simulink model "Driveline"  (R2020a)
settings: Solver=ode23tb  StartTime=0.0  StopTime=inf  FixedStep=.001  RelTol=1e-3
model workspace (MAT data in the model file):
  Trans.InputShaftInertia = 0.01
  Trans.InputShaftDamping = 0.001
  Trans.FinalDrive = 2.77
  Trans.GearRatios = [-3.82 4.56 4.56 2.97 2.08 1.69 1.27 1 0.85 0.65]
  Trans.GearNums = [-1 0 1 2 3 4 5 6 7 8]
  Trans.Inertias = [0.128 0.128 0.128 0.1 0.062 0.028 0.01 0.01 0.01 0.01]
  Trans.DampingCoeffs = [0.003 0.001 0.003 0.0025 0.002 0.001 0.001 0.001 0.001 0.001]
  Trans.Efficiencies = [0.9 0.9 0.9 0.9 0.9 0.95 0.95 0.95 0.95 0.95]
  Trans.ShiftTau = 0.02
  VEH.Mass = 330
  VEH.StaticNormalFrontLoad.FR = 74.25
  VEH.StaticNormalFrontLoad.FL = 74.25
  VEH.StaticNormalRearLoad.RR = 90.75
  VEH.StaticNormalRearLoad.RL = 90.75
  VEH.WheelBase = 1.575
  VEH.FrontAxlePositionfromCG = 0.847
  VEH.RearAxlePositionfromCG = 0.693
  VEH.HeightCG = 0.277
  VEH.FrontalArea = 1.435
  VEH.DragCoefficient = 0.33
  VEH.NumberOfWheelsPerAxle = 2
  VEH.Thread.FR = 1.705
  VEH.Thread.RR = 1.705
  VEH.PitchMomentInertia = 206
  VEH.RollMomentInertia = 206.613792
  VEH.YawMomentInertia = 206.613792
  VEH.SteeringRatio = 5.2
  VEH.TrackWidth = 1.2
  VEH.SprungMass = 290
  VEH.InitialLongPosition = 0
  VEH.InitialLatPosition = 0
  VEH.InitialVertPosition = 0
  VEH.InitialRollAngle = 0
  VEH.InitialPitchAngle = 0
  VEH.InitialYawAngle = 0
  VEH.InitialLongVel = 0
  VEH.InitialLatVel = 0
  VEH.InitialVertVel = 0
  VEH.InitialRollRate = 0
  VEH.InitialPitchRate = 0
  VEH.InitialYawRate = 0
  VEH.LongitudinalDragCoefficient = 1.06
  VEH.LongitudinalLCoefficient = -2.05
libraries: autolibsharedcoupling x4, vehdynlibsteering x1
settings Model: ModifiedByFormat=The MathWorks, Inc.  OrderedModelArguments=off  Creator=The MathWorks, Inc.  LastModifiedBy=The MathWorks, Inc.
settings SolverCC: ZeroCrossControl=DisableAll  DecoupledContinuousIntegration=on
settings DataIOCC: ReturnWorkspaceOutputs=off
settings DebuggingCC: ArtificialAlgebraicLoopMsg=none  IgnoredZcDiagnostic=none  PregeneratedLibrarySubsystemCodeDiagnostic=none  ArithmeticOperatorsInVariantConditions=warning
settings ModelReferenceCC: ModelReferenceMinAlgLoopOccurrences=on
settings SFSimCC: SimUseLocalCustomCode=off  CustomCodeUndefinedFunction=UseInterfaceOnly
settings RTWCC: RTWUseLocalCustomCode=off

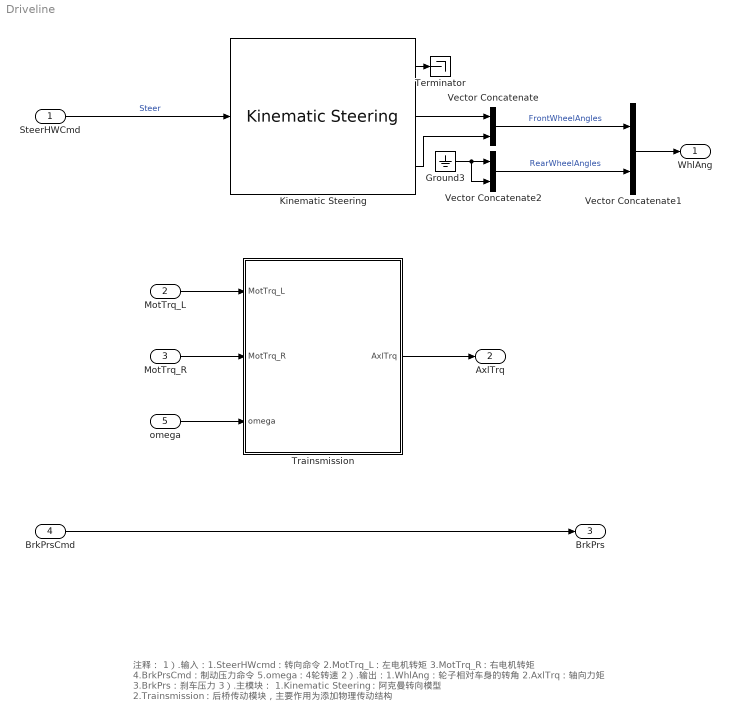
== system Driveline ==
  note: 注释：
      | 1）.输入：1.SteerHWcmd：转向命令
      | 2.MotTrq_L：左电机转矩
      | 3.MotTrq_R：右电机转矩
      | 4.BrkPrsCmd：制动压力命令
      | 5.omega：4轮转速
      | 2）.输出：1.WhlAng：轮子相对车身的转角
      | 2.AxlTrq：轴向力矩
      | 3.BrkPrs：刹车压力
      | 3）.主模块：
      | 1.Kinematic Steering：阿克曼转向模型
      | 2.Trainsmission：后桥传动模块，主要作用为添加物理传动结构
  SteerHWCmd : Inport
  MotTrq_L : Inport  Port=2
  MotTrq_R : Inport  Port=3
  BrkPrsCmd : Inport  Port=4  PortDimensions=4
  omega : Inport  Port=5
  Ground3 : Ground
  Kinematic Steering : vehdynlibsteering/Kinematic Steering  StrgType=Ackerman  StrgRatioType=Constant  Loc=Front  NrmlFctr=1  TrckWdth=VEH.WheelBase  WhlBase=(1.515+1.504)  Db=0  StrgRng=3*pi  StrgAngBpts="[-6.2832   -5.0265   -3.7699   -2.5133   -1.2566         0    1.2566    2.5133    3.7699    5.0265    6.2832]"  StrgRatioTbl=|  StrgRatio=5.2  StrgArmLngth=0.1  RckCsLngth=0.5  TieRodLngth=0.248128028933392  D=0.2  PnnRadius=0.0057  PnnRadiusTbl="[0.0055    0.0055    0.0056    0.0057    0.0057    0.0057    0.0057    0.0057    0.0056    0.0055    0.0055]"  RodLngth=0.1  ParaArmLngth=0.9  aMode=2
      | [13.5000   13.3750   13.2500   13.1250   13.0000   13.0000   13.0000   13.1250   13.2500   13.3750   13.5000
      | ]
      settings: SourceProductName=Vehicle Dynamics Blockset
  Terminator : Terminator
  Trainsmission : Subsystem
  Vector Concatenate : Concatenate
  Vector Concatenate1 : Concatenate
  Vector Concatenate2 : Concatenate
  WhlAng : Outport  Unit=rad  VectorParamsAs1DForOutWhenUnconnected=off
  AxlTrq : Outport  Port=2  VectorParamsAs1DForOutWhenUnconnected=off
  BrkPrs : Outport  Port=3  PortDimensions=4  VectorParamsAs1DForOutWhenUnconnected=off
  wires:
  Vector Concatenate1/1 -> WhlAng/1
  Vector Concatenate2/1 -> Vector Concatenate1/2  "RearWheelAngles"
  SteerHWCmd/1 -> Kinematic Steering/1  "Steer"
  Ground3/1 -> Vector Concatenate2/2, Vector Concatenate2/1
  Kinematic Steering/1 -> Terminator/1
  Kinematic Steering/3 -> Vector Concatenate/2
  Kinematic Steering/2 -> Vector Concatenate/1
  Vector Concatenate/1 -> Vector Concatenate1/1  "FrontWheelAngles"
  BrkPrsCmd/1 -> BrkPrs/1
  MotTrq_L/1 -> Trainsmission/1(MotTrq_L)
  MotTrq_R/1 -> Trainsmission/2(MotTrq_R)
  omega/1 -> Trainsmission/3(omega)
  Trainsmission/1(AxlTrq) -> AxlTrq/1

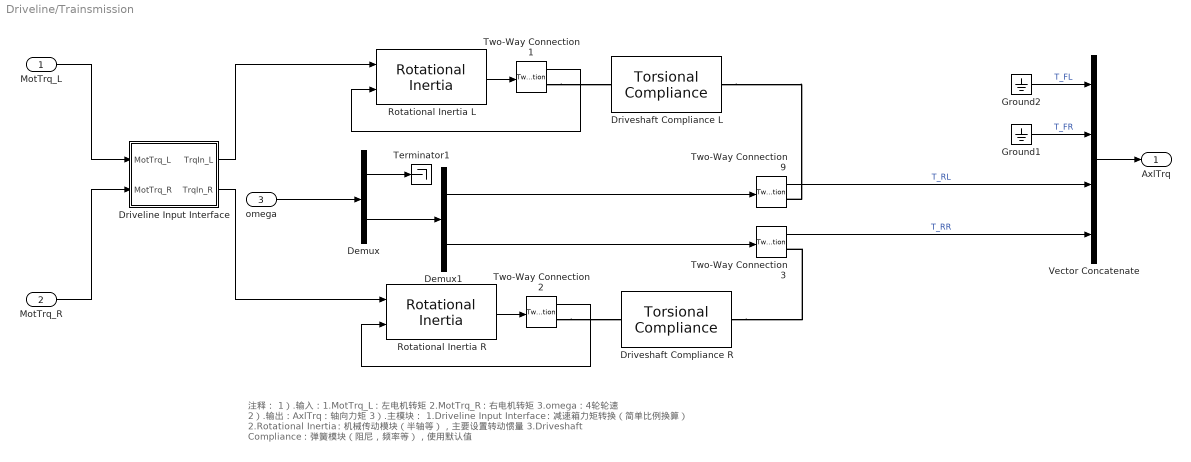
== system Driveline/Trainsmission ==
  note: 注释：
      | 1）.输入：1.MotTrq_L：左电机转矩
      | 2.MotTrq_R：右电机转矩
      | 3.omega：4轮轮速
      | 2）.输出：AxlTrq：轴向力矩
      | 3）.主模块：
      | 1.Driveline Input Interface：减速箱力矩转换（简单比例换算）
      | 2.Rotational Inertia：机械传动模块（半轴等），主要设置转动惯量
      | 3.Driveshaft Compliance：弹簧模块（阻尼，频率等），使用默认值
  MotTrq_L : Inport
  MotTrq_R : Inport  Port=2
  omega : Inport  Port=3
  Demux : Demux  Outputs=[2,2]
  Demux1 : Demux  Outputs=2
  Driveline Input Interface : Subsystem
  Driveshaft Compliance L : autolibsharedcoupling/Torsional Compliance  port_config=Two-way connection  extInfo=off  k=1000  b=10  theta_o=0  domega_o=0  omega_c=0.1  blkID=0  aMode=1
      settings: SourceProductBaseCode=PW,MT,VE,VP
  Driveshaft Compliance R : autolibsharedcoupling/Torsional Compliance  port_config=Two-way connection  extInfo=off  k=1000  b=10  theta_o=0  domega_o=0  omega_c=0.1  blkID=0  aMode=1
      settings: SourceProductBaseCode=PW,MT,VE,VP
  Ground1 : Ground
  Ground2 : Ground
  Rotational Inertia L : autolibsharedcoupling/Rotational Inertia  port_config=Simulink  extInfo=off  externJ=off  J=0.025887  b=.001  omega_o=0  blkID=0  aMode=1
      settings: SourceProductBaseCode=PW,MT,VE,VP
  Rotational Inertia R : autolibsharedcoupling/Rotational Inertia  port_config=Simulink  extInfo=off  externJ=off  J=0.025887  b=.001  omega_o=0  blkID=0  aMode=1
      settings: SourceProductBaseCode=PW,MT,VE,VP
  Terminator1 : Terminator
  Two-Way Connection{1..3,9} (4 alike) : TwoWayConnection
  Vector Concatenate : Concatenate  NumInputs=4
  AxlTrq : Outport  VectorParamsAs1DForOutWhenUnconnected=off
  wires:
  omega/1 -> Demux/1
  Ground2/1 -> Vector Concatenate/1  "T_FL"
  Demux1/2 -> Two-Way Connection3/1
  Vector Concatenate/1 -> AxlTrq/1
  MotTrq_L/1 -> Driveline Input Interface/1(MotTrq_L)
  Driveline Input Interface/1(TrqIn_L) -> Rotational Inertia L/1
  Two-Way Connection1/1 -> Rotational Inertia L/2
  Rotational Inertia L/1 -> Two-Way Connection1/1
  Two-Way Connection2/1 -> Rotational Inertia R/2
  Two-Way Connection3/1 -> Vector Concatenate/4  "T_RR"
  Demux/2 -> Demux1/1
  Driveline Input Interface/2(TrqIn_R) -> Rotational Inertia R/1
  Demux/1 -> Terminator1/1
  Ground1/1 -> Vector Concatenate/2  "T_FR"
  Two-Way Connection9/1 -> Vector Concatenate/3  "T_RL"
  MotTrq_R/1 -> Driveline Input Interface/2(MotTrq_R)
  Demux1/1 -> Two-Way Connection9/1
  Rotational Inertia R/1 -> Two-Way Connection2/1
  connections:
  Driveshaft Compliance L/RConn1 -- Two-Way Connection9/RConn1
  Two-Way Connection1/RConn1 -- Driveshaft Compliance L/LConn1
  Driveshaft Compliance R/RConn1 -- Two-Way Connection3/RConn1
  Two-Way Connection2/RConn1 -- Driveshaft Compliance R/LConn1

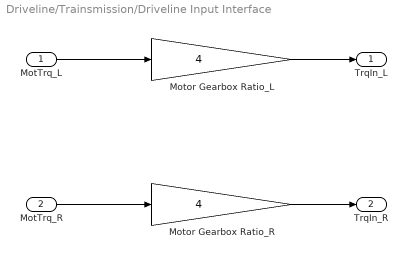
== system Driveline/Trainsmission/Driveline Input Interface ==
  MotTrq_L : Inport
  MotTrq_R : Inport  Port=2
  Motor Gearbox Ratio_L : Gain  Gain=4
  Motor Gearbox Ratio_R : Gain  Gain=4
  TrqIn_L : Outport  VectorParamsAs1DForOutWhenUnconnected=off
  TrqIn_R : Outport  Port=2  VectorParamsAs1DForOutWhenUnconnected=off
  wires:
  MotTrq_L/1 -> Motor Gearbox Ratio_L/1
  Motor Gearbox Ratio_L/1 -> TrqIn_L/1
  Motor Gearbox Ratio_R/1 -> TrqIn_R/1
  MotTrq_R/1 -> Motor Gearbox Ratio_R/1
